simulink model "Grid_SensorLayout_SpatialAllignment_Clustering"  (R2018a)
settings: Solver=FixedStepAuto  StartTime=0.0  StopTime=SimulationTime  FixedStep=SamplingTime  RelTol=1e-3
values from neighbouring files (symbols this model uses):
  ValidateGRID = true    [SensorFusion_Script0_main.m]
  ValidateLAYOUT = true    [SensorFusion_Script0_main.m]
  VisualizeCLUSTERING = true    [SensorFusion_Script0_main.m]
undefined symbols (not defined in the file or in its folder): ACTIVATE_CAM, ACTIVATE_RAD, CAM1_detTimeStamp, CAM1_MeasNoise, CAM1_objClassID, CAM1_PX, CAM1_PY, CAM1_VX, CAM1_VY, CAM2_detTimeStamp, CAM2_MeasNoise, CAM2_objClassID, CAM2_PX, CAM2_PY, CAM2_VX, CAM2_VY, CAM3_detTimeStamp, CAM3_MeasNoise, CAM3_objClassID, CAM3_PX, CAM3_PY, CAM3_VX, CAM3_VY, CAM4_detTimeStamp, CAM4_MeasNoise, CAM4_objClassID, CAM4_PX, CAM4_PY, CAM4_VX, CAM4_VY, CAM5_detTimeStamp, CAM5_MeasNoise, CAM5_objClassID, CAM5_PX, CAM5_PY, CAM5_VX, CAM5_VY, CAM6_detTimeStamp, CAM6_MeasNoise, CAM6_objClassID, CAM6_PX, CAM6_PY, CAM6_VX, CAM6_VY, CAM7_detTimeStamp, CAM7_MeasNoise, CAM7_objClassID, CAM7_PX, CAM7_PY, CAM7_VX, CAM7_VY, CAM8_detTimeStamp, CAM8_MeasNoise, CAM8_objClassID, CAM8_PX, CAM8_PY, CAM8_VX, CAM8_VY, CAM_nMeas, CAM_TYPE ... (+171)
libraries: simulink_extras x4
(part 5 of 10)

== system Grid_SensorLayout_SpatialAllignment_Clustering/SENSOR_MEASUREMENTS/RADAR_CAMERA_EGO_SENSOR_INTERFACE/CameraSensors/Camera5/ExtractMeasParam1 ==
  idx : Inport
  time : Inport  Port=2
  Constant : Constant  Value=CAM5_PX
  Constant1 : Constant  Value=CAM5_PY
  Constant2 : Constant  Value=CAM5_VX
  Constant3 : Constant  Value=CAM5_VY
  Constant4 : Constant  Value=CAM5_objClassID
  Constant5 : Constant  Value=CAM5_MeasNoise
  Constant6 : Constant  Value=CAM5_detTimeStamp
  Data Type Conversion : DataTypeConversion  OutDataTypeStr=int16
  MeasNoise : Selector  NumberOfDimensions=4  InputPortWidth=3  IndexOptions=Index vector (port),Select all,Select all,Index vector (port)  Indices=[1 3],1,1,1  OutputSizes=1,1,1,1
  PosX : Selector  NumberOfDimensions=2  InputPortWidth=3  IndexOptions=Index vector (port),Index vector (port)  Indices=[1 3],1  OutputSizes=1,1
  PosY : Selector  NumberOfDimensions=2  InputPortWidth=3  IndexOptions=Index vector (port),Index vector (port)  Indices=[1 3],1  OutputSizes=1,1
  Reshape : Reshape  OutputDimensionality=Customize  OutputDimensions=[4,4]
  VelX : Selector  NumberOfDimensions=2  InputPortWidth=3  IndexOptions=Index vector (port),Index vector (port)  Indices=[1 3],1  OutputSizes=1,1
  VelY : Selector  NumberOfDimensions=2  InputPortWidth=3  IndexOptions=Index vector (port),Index vector (port)  Indices=[1 3],1  OutputSizes=1,1
  snr : Selector  NumberOfDimensions=2  InputPortWidth=3  IndexOptions=Index vector (port),Index vector (port)  Indices=[1 3],1  OutputSizes=1,1
  timeStamp : Selector  NumberOfDimensions=2  InputPortWidth=3  IndexOptions=Select all,Index vector (port)  Indices=[1 3],1  OutputSizes=1,1
  PX : Outport
  PY : Outport  Port=2
  VX : Outport  Port=3
  VY : Outport  Port=4
  OBJ_TYPE : Outport  Port=5
  NOISE_COV : Outport  Port=6
  measCaptureTime : Outport  Port=7
  wires:
  Constant3/1 -> VelY/1
  Constant2/1 -> VelX/1
  VelY/1 -> VY/1
  Constant/1 -> PosX/1
  idx/1 -> MeasNoise/3, snr/3, VelY/3, VelX/3, PosY/3, PosX/3
  Constant1/1 -> PosY/1
  VelX/1 -> VX/1
  PosX/1 -> PX/1
  PosY/1 -> PY/1
  time/1 -> timeStamp/2, MeasNoise/2, snr/2, VelY/2, VelX/2, PosY/2, PosX/2
  Constant4/1 -> snr/1
  snr/1 -> Data Type Conversion/1
  Constant5/1 -> MeasNoise/1
  Constant6/1 -> timeStamp/1
  MeasNoise/1 -> Reshape/1
  timeStamp/1 -> measCaptureTime/1
  Reshape/1 -> NOISE_COV/1
  Data Type Conversion/1 -> OBJ_TYPE/1

== system Grid_SensorLayout_SpatialAllignment_Clustering/SENSOR_MEASUREMENTS/RADAR_CAMERA_EGO_SENSOR_INTERFACE/CameraSensors/Camera5/IsValid2 ==
  idx : Inport
  px : Inport  Port=2
  py : Inport  Port=3
  vx : Inport  Port=4
  vy : Inport  Port=5
  Abs{,1..3} (4 alike) : Abs
  Add : Sum  Inputs=++++
  Constant : Constant  Value=uint16(0)
  Data Type Conversion : DataTypeConversion  OutDataTypeStr=uint16
  Switch : Switch  Threshold=0.0001
  ID : Outport
  wires:
  Add/1 -> Switch/2
  Abs2/1 -> Add/3
  Constant/1 -> Switch/3
  Abs/1 -> Add/1
  px/1 -> Abs/1
  Abs3/1 -> Add/4
  Abs1/1 -> Add/2
  vy/1 -> Abs3/1
  py/1 -> Abs1/1
  vx/1 -> Abs2/1
  idx/1 -> Data Type Conversion/1
  Switch/1 -> ID/1
  Data Type Conversion/1 -> Switch/1

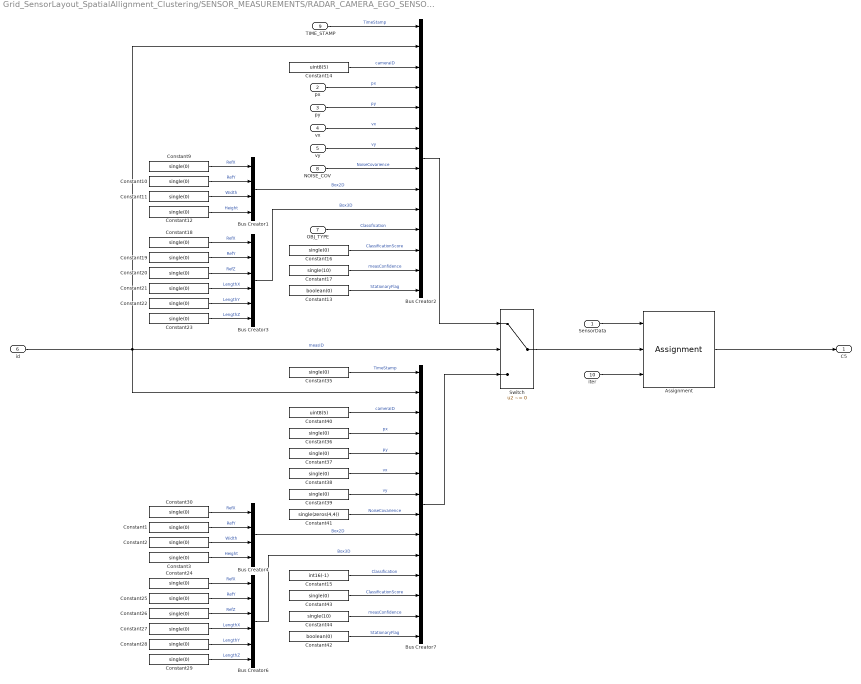
== system Grid_SensorLayout_SpatialAllignment_Clustering/SENSOR_MEASUREMENTS/RADAR_CAMERA_EGO_SENSOR_INTERFACE/CameraSensors/Camera5/Subsystem1 ==
  SensorData : Inport
  px : Inport  Port=2
  py : Inport  Port=3
  vx : Inport  Port=4
  vy : Inport  Port=5
  id : Inport  Port=6
  OBJ_TYPE : Inport  Port=7
  NOISE_COV : Inport  Port=8
  TIME_STAMP : Inport  Port=9
  iter : Inport  Port=10
  Assignment : Assignment  DiagnosticForDimensions=Warning  IndexOptions=Index vector (port)  Indices=1  OutputSizes=1
  Bus Creator1 : BusCreator  Inputs=4  OutDataTypeStr=Bus: BoxParam2D  NonVirtualBus=on
  Bus Creator2 : BusCreator  Inputs=14  OutDataTypeStr=Bus: CameraMeasParam  NonVirtualBus=on
  Bus Creator3 : BusCreator  Inputs=6  OutDataTypeStr=Bus: BoxParam3D  NonVirtualBus=on
  Bus Creator4 : BusCreator  Inputs=4  OutDataTypeStr=Bus: BoxParam2D  NonVirtualBus=on
  Bus Creator6 : BusCreator  Inputs=6  OutDataTypeStr=Bus: BoxParam3D  NonVirtualBus=on
  Bus Creator7 : BusCreator  Inputs=14  OutDataTypeStr=Bus: CameraMeasParam  NonVirtualBus=on
  Constant{1..3,9..12,16,18..30,35..39,43} (27 alike) : Constant  Value=single(0)
  Constant13 : Constant  Value=boolean(0)
  Constant14 : Constant  Value=uint8(5)
  Constant15 : Constant  Value=int16(-1)
  Constant17 : Constant  Value=single(10)
  Constant40 : Constant  Value=uint8(5)
  Constant41 : Constant  Value=single(zeros(4,4))
  Constant42 : Constant  Value=boolean(0)
  Constant44 : Constant  Value=single(10)
  Switch : Switch  Criteria=u2 ~= 0
  C5 : Outport
  wires:
  Bus Creator4/1 -> Bus Creator7/9  "Box2D"
  Bus Creator1/1 -> Bus Creator2/9  "Box2D"
  Bus Creator7/1 -> Switch/3
  Constant3/1 -> Bus Creator4/4  "Height"
  Constant44/1 -> Bus Creator7/13  "measConfidence"
  Constant19/1 -> Bus Creator3/2  "RefY"
  id/1 -> Bus Creator7/2, Bus Creator2/2, Switch/2  "measID"
  Bus Creator2/1 -> Switch/1
  Constant2/1 -> Bus Creator4/3  "Width"
  Constant12/1 -> Bus Creator1/4  "Height"
  Constant43/1 -> Bus Creator7/12  "ClassificationScore"
  Constant41/1 -> Bus Creator7/8  "NoiseCovarience"
  Constant20/1 -> Bus Creator3/3  "RefZ"
  Constant37/1 -> Bus Creator7/5  "py"
  Constant23/1 -> Bus Creator3/6  "LengthZ"
  Constant11/1 -> Bus Creator1/3  "Width"
  Constant18/1 -> Bus Creator3/1  "RefX"
  Constant9/1 -> Bus Creator1/1  "RefX"
  Constant27/1 -> Bus Creator6/4  "LengthX"
  Bus Creator3/1 -> Bus Creator2/10  "Box3D"
  Constant17/1 -> Bus Creator2/13  "measConfidence"
  py/1 -> Bus Creator2/5  "py"
  Constant36/1 -> Bus Creator7/4  "px"
  Constant16/1 -> Bus Creator2/12  "ClassificationScore"
  Constant42/1 -> Bus Creator7/14  "StationaryFlag"
  SensorData/1 -> Assignment/1
  px/1 -> Bus Creator2/4  "px"
  Constant39/1 -> Bus Creator7/7  "vy"
  Constant35/1 -> Bus Creator7/1  "TimeStamp"
  Constant38/1 -> Bus Creator7/6  "vx"
  TIME_STAMP/1 -> Bus Creator2/1  "TimeStamp"
  Switch/1 -> Assignment/2
  iter/1 -> Assignment/3
  Bus Creator6/1 -> Bus Creator7/10  "Box3D"
  Constant10/1 -> Bus Creator1/2  "RefY"
  NOISE_COV/1 -> Bus Creator2/8  "NoiseCovarience"
  Constant21/1 -> Bus Creator3/4  "LengthX"
  Constant1/1 -> Bus Creator4/2  "RefY"
  Constant25/1 -> Bus Creator6/2  "RefY"
  Constant26/1 -> Bus Creator6/3  "RefZ"
  Constant29/1 -> Bus Creator6/6  "LengthZ"
  Constant30/1 -> Bus Creator4/1  "RefX"
  vx/1 -> Bus Creator2/6  "vx"
  Constant13/1 -> Bus Creator2/14  "StationaryFlag"
  Constant22/1 -> Bus Creator3/5  "LengthY"
  Constant24/1 -> Bus Creator6/1  "RefX"
  Constant40/1 -> Bus Creator7/3  "cameraID"
  Constant28/1 -> Bus Creator6/5  "LengthY"
  Assignment/1 -> C5/1
  Constant15/1 -> Bus Creator7/11  "Classification"
  Constant14/1 -> Bus Creator2/3  "cameraID"
  vy/1 -> Bus Creator2/7  "vy"
  OBJ_TYPE/1 -> Bus Creator2/11  "Classification"

== system Grid_SensorLayout_SpatialAllignment_Clustering/SENSOR_MEASUREMENTS/RADAR_CAMERA_EGO_SENSOR_INTERFACE/CameraSensors/Camera6/ExtractMeasParam1 ==
  idx : Inport
  time : Inport  Port=2
  Constant : Constant  Value=CAM6_PX
  Constant1 : Constant  Value=CAM6_PY
  Constant2 : Constant  Value=CAM6_VX
  Constant3 : Constant  Value=CAM6_VY
  Constant4 : Constant  Value=CAM6_objClassID
  Constant5 : Constant  Value=CAM6_MeasNoise
  Constant6 : Constant  Value=CAM6_detTimeStamp
  Data Type Conversion : DataTypeConversion  OutDataTypeStr=int16
  MeasNoise : Selector  NumberOfDimensions=4  InputPortWidth=3  IndexOptions=Index vector (port),Select all,Select all,Index vector (port)  Indices=[1 3],1,1,1  OutputSizes=1,1,1,1
  PosX : Selector  NumberOfDimensions=2  InputPortWidth=3  IndexOptions=Index vector (port),Index vector (port)  Indices=[1 3],1  OutputSizes=1,1
  PosY : Selector  NumberOfDimensions=2  InputPortWidth=3  IndexOptions=Index vector (port),Index vector (port)  Indices=[1 3],1  OutputSizes=1,1
  Reshape : Reshape  OutputDimensionality=Customize  OutputDimensions=[4,4]
  VelX : Selector  NumberOfDimensions=2  InputPortWidth=3  IndexOptions=Index vector (port),Index vector (port)  Indices=[1 3],1  OutputSizes=1,1
  VelY : Selector  NumberOfDimensions=2  InputPortWidth=3  IndexOptions=Index vector (port),Index vector (port)  Indices=[1 3],1  OutputSizes=1,1
  snr : Selector  NumberOfDimensions=2  InputPortWidth=3  IndexOptions=Index vector (port),Index vector (port)  Indices=[1 3],1  OutputSizes=1,1
  timeStamp : Selector  NumberOfDimensions=2  InputPortWidth=3  IndexOptions=Select all,Index vector (port)  Indices=[1 3],1  OutputSizes=1,1
  PX : Outport
  PY : Outport  Port=2
  VX : Outport  Port=3
  VY : Outport  Port=4
  OBJ_TYPE : Outport  Port=5
  NOISE_COV : Outport  Port=6
  measCaptureTime : Outport  Port=7
  wires:
  Constant3/1 -> VelY/1
  Constant2/1 -> VelX/1
  VelY/1 -> VY/1
  Constant/1 -> PosX/1
  idx/1 -> MeasNoise/3, snr/3, VelY/3, VelX/3, PosY/3, PosX/3
  Constant1/1 -> PosY/1
  VelX/1 -> VX/1
  PosX/1 -> PX/1
  PosY/1 -> PY/1
  time/1 -> timeStamp/2, MeasNoise/2, snr/2, VelY/2, VelX/2, PosY/2, PosX/2
  Constant4/1 -> snr/1
  snr/1 -> Data Type Conversion/1
  Constant5/1 -> MeasNoise/1
  Constant6/1 -> timeStamp/1
  MeasNoise/1 -> Reshape/1
  timeStamp/1 -> measCaptureTime/1
  Reshape/1 -> NOISE_COV/1
  Data Type Conversion/1 -> OBJ_TYPE/1

== system Grid_SensorLayout_SpatialAllignment_Clustering/SENSOR_MEASUREMENTS/RADAR_CAMERA_EGO_SENSOR_INTERFACE/CameraSensors/Camera6/IsValid2 ==
  idx : Inport
  px : Inport  Port=2
  py : Inport  Port=3
  vx : Inport  Port=4
  vy : Inport  Port=5
  Abs{,1..3} (4 alike) : Abs
  Add : Sum  Inputs=++++
  Constant : Constant  Value=uint16(0)
  Data Type Conversion : DataTypeConversion  OutDataTypeStr=uint16
  Switch : Switch  Threshold=0.0001
  ID : Outport
  wires:
  Add/1 -> Switch/2
  Abs2/1 -> Add/3
  Constant/1 -> Switch/3
  Abs/1 -> Add/1
  px/1 -> Abs/1
  Abs3/1 -> Add/4
  Abs1/1 -> Add/2
  vy/1 -> Abs3/1
  py/1 -> Abs1/1
  vx/1 -> Abs2/1
  idx/1 -> Data Type Conversion/1
  Switch/1 -> ID/1
  Data Type Conversion/1 -> Switch/1

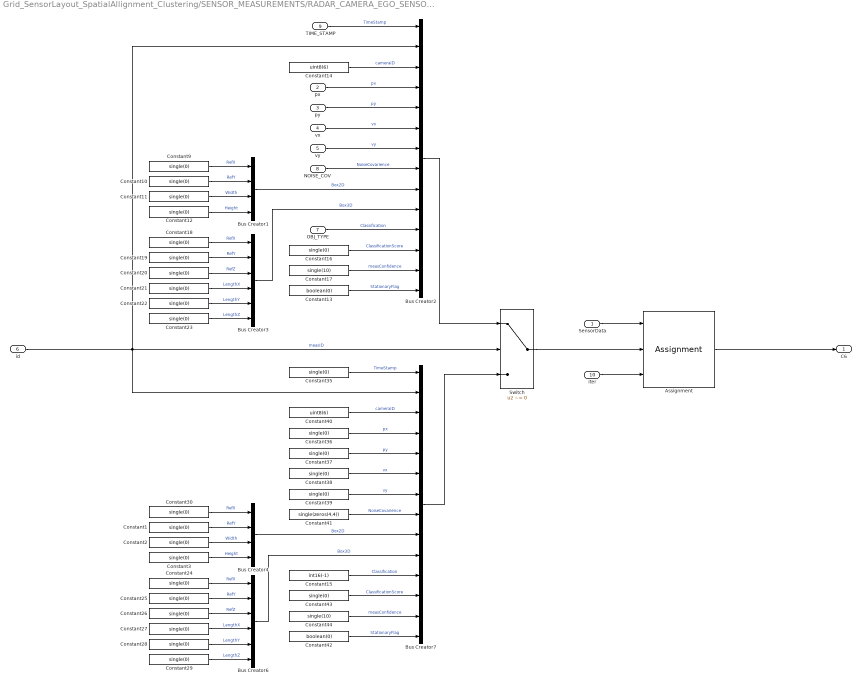
== system Grid_SensorLayout_SpatialAllignment_Clustering/SENSOR_MEASUREMENTS/RADAR_CAMERA_EGO_SENSOR_INTERFACE/CameraSensors/Camera6/Subsystem1 ==
  SensorData : Inport
  px : Inport  Port=2
  py : Inport  Port=3
  vx : Inport  Port=4
  vy : Inport  Port=5
  id : Inport  Port=6
  OBJ_TYPE : Inport  Port=7
  NOISE_COV : Inport  Port=8
  TIME_STAMP : Inport  Port=9
  iter : Inport  Port=10
  Assignment : Assignment  DiagnosticForDimensions=Warning  IndexOptions=Index vector (port)  Indices=1  OutputSizes=1
  Bus Creator1 : BusCreator  Inputs=4  OutDataTypeStr=Bus: BoxParam2D  NonVirtualBus=on
  Bus Creator2 : BusCreator  Inputs=14  OutDataTypeStr=Bus: CameraMeasParam  NonVirtualBus=on
  Bus Creator3 : BusCreator  Inputs=6  OutDataTypeStr=Bus: BoxParam3D  NonVirtualBus=on
  Bus Creator4 : BusCreator  Inputs=4  OutDataTypeStr=Bus: BoxParam2D  NonVirtualBus=on
  Bus Creator6 : BusCreator  Inputs=6  OutDataTypeStr=Bus: BoxParam3D  NonVirtualBus=on
  Bus Creator7 : BusCreator  Inputs=14  OutDataTypeStr=Bus: CameraMeasParam  NonVirtualBus=on
  Constant{1..3,9..12,16,18..30,35..39,43} (27 alike) : Constant  Value=single(0)
  Constant13 : Constant  Value=boolean(0)
  Constant14 : Constant  Value=uint8(6)
  Constant15 : Constant  Value=int16(-1)
  Constant17 : Constant  Value=single(10)
  Constant40 : Constant  Value=uint8(6)
  Constant41 : Constant  Value=single(zeros(4,4))
  Constant42 : Constant  Value=boolean(0)
  Constant44 : Constant  Value=single(10)
  Switch : Switch  Criteria=u2 ~= 0
  C6 : Outport
  wires:
  Bus Creator4/1 -> Bus Creator7/9  "Box2D"
  Bus Creator1/1 -> Bus Creator2/9  "Box2D"
  Bus Creator7/1 -> Switch/3
  Constant3/1 -> Bus Creator4/4  "Height"
  Constant44/1 -> Bus Creator7/13  "measConfidence"
  Constant19/1 -> Bus Creator3/2  "RefY"
  id/1 -> Bus Creator7/2, Bus Creator2/2, Switch/2  "measID"
  Bus Creator2/1 -> Switch/1
  Constant2/1 -> Bus Creator4/3  "Width"
  Constant12/1 -> Bus Creator1/4  "Height"
  Constant43/1 -> Bus Creator7/12  "ClassificationScore"
  Constant41/1 -> Bus Creator7/8  "NoiseCovarience"
  Constant20/1 -> Bus Creator3/3  "RefZ"
  Constant37/1 -> Bus Creator7/5  "py"
  Constant23/1 -> Bus Creator3/6  "LengthZ"
  Constant11/1 -> Bus Creator1/3  "Width"
  Constant18/1 -> Bus Creator3/1  "RefX"
  Constant9/1 -> Bus Creator1/1  "RefX"
  Constant27/1 -> Bus Creator6/4  "LengthX"
  Bus Creator3/1 -> Bus Creator2/10  "Box3D"
  Constant17/1 -> Bus Creator2/13  "measConfidence"
  py/1 -> Bus Creator2/5  "py"
  Constant36/1 -> Bus Creator7/4  "px"
  Constant16/1 -> Bus Creator2/12  "ClassificationScore"
  Constant42/1 -> Bus Creator7/14  "StationaryFlag"
  SensorData/1 -> Assignment/1
  px/1 -> Bus Creator2/4  "px"
  Constant39/1 -> Bus Creator7/7  "vy"
  Constant35/1 -> Bus Creator7/1  "TimeStamp"
  Constant38/1 -> Bus Creator7/6  "vx"
  TIME_STAMP/1 -> Bus Creator2/1  "TimeStamp"
  Switch/1 -> Assignment/2
  iter/1 -> Assignment/3
  Bus Creator6/1 -> Bus Creator7/10  "Box3D"
  Constant10/1 -> Bus Creator1/2  "RefY"
  NOISE_COV/1 -> Bus Creator2/8  "NoiseCovarience"
  Constant21/1 -> Bus Creator3/4  "LengthX"
  Constant1/1 -> Bus Creator4/2  "RefY"
  Constant25/1 -> Bus Creator6/2  "RefY"
  Constant26/1 -> Bus Creator6/3  "RefZ"
  Constant29/1 -> Bus Creator6/6  "LengthZ"
  Constant30/1 -> Bus Creator4/1  "RefX"
  vx/1 -> Bus Creator2/6  "vx"
  Constant13/1 -> Bus Creator2/14  "StationaryFlag"
  Constant22/1 -> Bus Creator3/5  "LengthY"
  Constant24/1 -> Bus Creator6/1  "RefX"
  Constant40/1 -> Bus Creator7/3  "cameraID"
  Constant28/1 -> Bus Creator6/5  "LengthY"
  Assignment/1 -> C6/1
  Constant15/1 -> Bus Creator7/11  "Classification"
  Constant14/1 -> Bus Creator2/3  "cameraID"
  vy/1 -> Bus Creator2/7  "vy"
  OBJ_TYPE/1 -> Bus Creator2/11  "Classification"

== system Grid_SensorLayout_SpatialAllignment_Clustering/SENSOR_MEASUREMENTS/RADAR_CAMERA_EGO_SENSOR_INTERFACE/CameraSensors/Camera7/ExtractMeasParam1 ==
  idx : Inport
  time : Inport  Port=2
  Constant : Constant  Value=CAM7_PX
  Constant1 : Constant  Value=CAM7_PY
  Constant2 : Constant  Value=CAM7_VX
  Constant3 : Constant  Value=CAM7_VY
  Constant4 : Constant  Value=CAM7_objClassID
  Constant5 : Constant  Value=CAM7_MeasNoise
  Constant6 : Constant  Value=CAM7_detTimeStamp
  Data Type Conversion : DataTypeConversion  OutDataTypeStr=int16
  MeasNoise : Selector  NumberOfDimensions=4  InputPortWidth=3  IndexOptions=Index vector (port),Select all,Select all,Index vector (port)  Indices=[1 3],1,1,1  OutputSizes=1,1,1,1
  PosX : Selector  NumberOfDimensions=2  InputPortWidth=3  IndexOptions=Index vector (port),Index vector (port)  Indices=[1 3],1  OutputSizes=1,1
  PosY : Selector  NumberOfDimensions=2  InputPortWidth=3  IndexOptions=Index vector (port),Index vector (port)  Indices=[1 3],1  OutputSizes=1,1
  Reshape : Reshape  OutputDimensionality=Customize  OutputDimensions=[4,4]
  VelX : Selector  NumberOfDimensions=2  InputPortWidth=3  IndexOptions=Index vector (port),Index vector (port)  Indices=[1 3],1  OutputSizes=1,1
  VelY : Selector  NumberOfDimensions=2  InputPortWidth=3  IndexOptions=Index vector (port),Index vector (port)  Indices=[1 3],1  OutputSizes=1,1
  snr : Selector  NumberOfDimensions=2  InputPortWidth=3  IndexOptions=Index vector (port),Index vector (port)  Indices=[1 3],1  OutputSizes=1,1
  timeStamp : Selector  NumberOfDimensions=2  InputPortWidth=3  IndexOptions=Select all,Index vector (port)  Indices=[1 3],1  OutputSizes=1,1
  PX : Outport
  PY : Outport  Port=2
  VX : Outport  Port=3
  VY : Outport  Port=4
  OBJ_TYPE : Outport  Port=5
  NOISE_COV : Outport  Port=6
  measCaptureTime : Outport  Port=7
  wires:
  Constant3/1 -> VelY/1
  Constant2/1 -> VelX/1
  VelY/1 -> VY/1
  Constant/1 -> PosX/1
  idx/1 -> MeasNoise/3, snr/3, VelY/3, VelX/3, PosY/3, PosX/3
  Constant1/1 -> PosY/1
  VelX/1 -> VX/1
  PosX/1 -> PX/1
  PosY/1 -> PY/1
  time/1 -> timeStamp/2, MeasNoise/2, snr/2, VelY/2, VelX/2, PosY/2, PosX/2
  Constant4/1 -> snr/1
  snr/1 -> Data Type Conversion/1
  Constant5/1 -> MeasNoise/1
  Constant6/1 -> timeStamp/1
  MeasNoise/1 -> Reshape/1
  timeStamp/1 -> measCaptureTime/1
  Reshape/1 -> NOISE_COV/1
  Data Type Conversion/1 -> OBJ_TYPE/1

== system Grid_SensorLayout_SpatialAllignment_Clustering/SENSOR_MEASUREMENTS/RADAR_CAMERA_EGO_SENSOR_INTERFACE/CameraSensors/Camera7/IsValid2 ==
  idx : Inport
  px : Inport  Port=2
  py : Inport  Port=3
  vx : Inport  Port=4
  vy : Inport  Port=5
  Abs{,1..3} (4 alike) : Abs
  Add : Sum  Inputs=++++
  Constant : Constant  Value=uint16(0)
  Data Type Conversion : DataTypeConversion  OutDataTypeStr=uint16
  Switch : Switch  Threshold=0.0001
  ID : Outport
  wires:
  Add/1 -> Switch/2
  Abs2/1 -> Add/3
  Constant/1 -> Switch/3
  Abs/1 -> Add/1
  px/1 -> Abs/1
  Abs3/1 -> Add/4
  Abs1/1 -> Add/2
  vy/1 -> Abs3/1
  py/1 -> Abs1/1
  vx/1 -> Abs2/1
  idx/1 -> Data Type Conversion/1
  Switch/1 -> ID/1
  Data Type Conversion/1 -> Switch/1

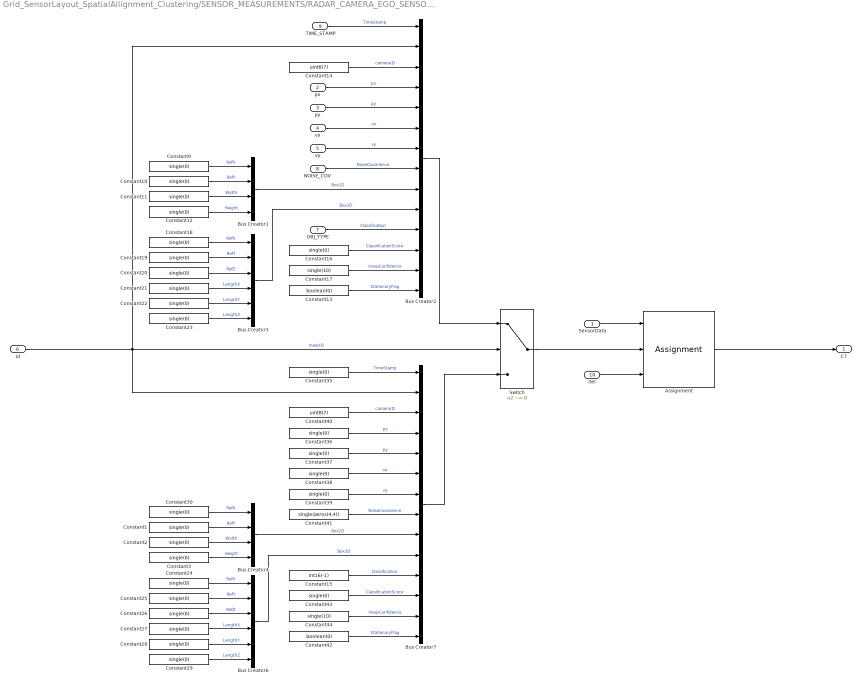
== system Grid_SensorLayout_SpatialAllignment_Clustering/SENSOR_MEASUREMENTS/RADAR_CAMERA_EGO_SENSOR_INTERFACE/CameraSensors/Camera7/Subsystem1 ==
  SensorData : Inport
  px : Inport  Port=2
  py : Inport  Port=3
  vx : Inport  Port=4
  vy : Inport  Port=5
  id : Inport  Port=6
  OBJ_TYPE : Inport  Port=7
  NOISE_COV : Inport  Port=8
  TIME_STAMP : Inport  Port=9
  iter : Inport  Port=10
  Assignment : Assignment  DiagnosticForDimensions=Warning  IndexOptions=Index vector (port)  Indices=1  OutputSizes=1
  Bus Creator1 : BusCreator  Inputs=4  OutDataTypeStr=Bus: BoxParam2D  NonVirtualBus=on
  Bus Creator2 : BusCreator  Inputs=14  OutDataTypeStr=Bus: CameraMeasParam  NonVirtualBus=on
  Bus Creator3 : BusCreator  Inputs=6  OutDataTypeStr=Bus: BoxParam3D  NonVirtualBus=on
  Bus Creator4 : BusCreator  Inputs=4  OutDataTypeStr=Bus: BoxParam2D  NonVirtualBus=on
  Bus Creator6 : BusCreator  Inputs=6  OutDataTypeStr=Bus: BoxParam3D  NonVirtualBus=on
  Bus Creator7 : BusCreator  Inputs=14  OutDataTypeStr=Bus: CameraMeasParam  NonVirtualBus=on
  Constant{1..3,9..12,16,18..30,35..39,43} (27 alike) : Constant  Value=single(0)
  Constant13 : Constant  Value=boolean(0)
  Constant14 : Constant  Value=uint8(7)
  Constant15 : Constant  Value=int16(-1)
  Constant17 : Constant  Value=single(10)
  Constant40 : Constant  Value=uint8(7)
  Constant41 : Constant  Value=single(zeros(4,4))
  Constant42 : Constant  Value=boolean(0)
  Constant44 : Constant  Value=single(10)
  Switch : Switch  Criteria=u2 ~= 0
  C7 : Outport
  wires:
  Bus Creator4/1 -> Bus Creator7/9  "Box2D"
  Bus Creator1/1 -> Bus Creator2/9  "Box2D"
  Bus Creator7/1 -> Switch/3
  Constant3/1 -> Bus Creator4/4  "Height"
  Constant44/1 -> Bus Creator7/13  "measConfidence"
  Constant19/1 -> Bus Creator3/2  "RefY"
  id/1 -> Bus Creator7/2, Bus Creator2/2, Switch/2  "measID"
  Bus Creator2/1 -> Switch/1
  Constant2/1 -> Bus Creator4/3  "Width"
  Constant12/1 -> Bus Creator1/4  "Height"
  Constant43/1 -> Bus Creator7/12  "ClassificationScore"
  Constant41/1 -> Bus Creator7/8  "NoiseCovarience"
  Constant20/1 -> Bus Creator3/3  "RefZ"
  Constant37/1 -> Bus Creator7/5  "py"
  Constant23/1 -> Bus Creator3/6  "LengthZ"
  Constant11/1 -> Bus Creator1/3  "Width"
  Constant18/1 -> Bus Creator3/1  "RefX"
  Constant9/1 -> Bus Creator1/1  "RefX"
  Constant27/1 -> Bus Creator6/4  "LengthX"
  Bus Creator3/1 -> Bus Creator2/10  "Box3D"
  Constant17/1 -> Bus Creator2/13  "measConfidence"
  py/1 -> Bus Creator2/5  "py"
  Constant36/1 -> Bus Creator7/4  "px"
  Constant16/1 -> Bus Creator2/12  "ClassificationScore"
  Constant42/1 -> Bus Creator7/14  "StationaryFlag"
  SensorData/1 -> Assignment/1
  px/1 -> Bus Creator2/4  "px"
  Constant39/1 -> Bus Creator7/7  "vy"
  Constant35/1 -> Bus Creator7/1  "TimeStamp"
  Constant38/1 -> Bus Creator7/6  "vx"
  TIME_STAMP/1 -> Bus Creator2/1  "TimeStamp"
  Switch/1 -> Assignment/2
  iter/1 -> Assignment/3
  Bus Creator6/1 -> Bus Creator7/10  "Box3D"
  Constant10/1 -> Bus Creator1/2  "RefY"
  NOISE_COV/1 -> Bus Creator2/8  "NoiseCovarience"
  Constant21/1 -> Bus Creator3/4  "LengthX"
  Constant1/1 -> Bus Creator4/2  "RefY"
  Constant25/1 -> Bus Creator6/2  "RefY"
  Constant26/1 -> Bus Creator6/3  "RefZ"
  Constant29/1 -> Bus Creator6/6  "LengthZ"
  Constant30/1 -> Bus Creator4/1  "RefX"
  vx/1 -> Bus Creator2/6  "vx"
  Constant13/1 -> Bus Creator2/14  "StationaryFlag"
  Constant22/1 -> Bus Creator3/5  "LengthY"
  Constant24/1 -> Bus Creator6/1  "RefX"
  Constant40/1 -> Bus Creator7/3  "cameraID"
  Constant28/1 -> Bus Creator6/5  "LengthY"
  Assignment/1 -> C7/1
  Constant15/1 -> Bus Creator7/11  "Classification"
  Constant14/1 -> Bus Creator2/3  "cameraID"
  vy/1 -> Bus Creator2/7  "vy"
  OBJ_TYPE/1 -> Bus Creator2/11  "Classification"

== system Grid_SensorLayout_SpatialAllignment_Clustering/SENSOR_MEASUREMENTS/RADAR_CAMERA_EGO_SENSOR_INTERFACE/CameraSensors/Camera8/ExtractMeasParam1 ==
  idx : Inport
  time : Inport  Port=2
  Constant : Constant  Value=CAM8_PX
  Constant1 : Constant  Value=CAM8_PY
  Constant2 : Constant  Value=CAM8_VX
  Constant3 : Constant  Value=CAM8_VY
  Constant4 : Constant  Value=CAM8_objClassID
  Constant5 : Constant  Value=CAM8_MeasNoise
  Constant6 : Constant  Value=CAM8_detTimeStamp
  Data Type Conversion : DataTypeConversion  OutDataTypeStr=int16
  MeasNoise : Selector  NumberOfDimensions=4  InputPortWidth=3  IndexOptions=Index vector (port),Select all,Select all,Index vector (port)  Indices=[1 3],1,1,1  OutputSizes=1,1,1,1
  PosX : Selector  NumberOfDimensions=2  InputPortWidth=3  IndexOptions=Index vector (port),Index vector (port)  Indices=[1 3],1  OutputSizes=1,1
  PosY : Selector  NumberOfDimensions=2  InputPortWidth=3  IndexOptions=Index vector (port),Index vector (port)  Indices=[1 3],1  OutputSizes=1,1
  Reshape : Reshape  OutputDimensionality=Customize  OutputDimensions=[4,4]
  VelX : Selector  NumberOfDimensions=2  InputPortWidth=3  IndexOptions=Index vector (port),Index vector (port)  Indices=[1 3],1  OutputSizes=1,1
  VelY : Selector  NumberOfDimensions=2  InputPortWidth=3  IndexOptions=Index vector (port),Index vector (port)  Indices=[1 3],1  OutputSizes=1,1
  snr : Selector  NumberOfDimensions=2  InputPortWidth=3  IndexOptions=Index vector (port),Index vector (port)  Indices=[1 3],1  OutputSizes=1,1
  timeStamp : Selector  NumberOfDimensions=2  InputPortWidth=3  IndexOptions=Select all,Index vector (port)  Indices=[1 3],1  OutputSizes=1,1
  PX : Outport
  PY : Outport  Port=2
  VX : Outport  Port=3
  VY : Outport  Port=4
  OBJ_TYPE : Outport  Port=5
  NOISE_COV : Outport  Port=6
  measCaptureTime : Outport  Port=7
  wires:
  Constant3/1 -> VelY/1
  Constant2/1 -> VelX/1
  VelY/1 -> VY/1
  Constant/1 -> PosX/1
  idx/1 -> MeasNoise/3, snr/3, VelY/3, VelX/3, PosY/3, PosX/3
  Constant1/1 -> PosY/1
  VelX/1 -> VX/1
  PosX/1 -> PX/1
  PosY/1 -> PY/1
  time/1 -> timeStamp/2, MeasNoise/2, snr/2, VelY/2, VelX/2, PosY/2, PosX/2
  Constant4/1 -> snr/1
  snr/1 -> Data Type Conversion/1
  Constant5/1 -> MeasNoise/1
  Constant6/1 -> timeStamp/1
  MeasNoise/1 -> Reshape/1
  timeStamp/1 -> measCaptureTime/1
  Reshape/1 -> NOISE_COV/1
  Data Type Conversion/1 -> OBJ_TYPE/1

== system Grid_SensorLayout_SpatialAllignment_Clustering/SENSOR_MEASUREMENTS/RADAR_CAMERA_EGO_SENSOR_INTERFACE/CameraSensors/Camera8/IsValid2 ==
  idx : Inport
  px : Inport  Port=2
  py : Inport  Port=3
  vx : Inport  Port=4
  vy : Inport  Port=5
  Abs{,1..3} (4 alike) : Abs
  Add : Sum  Inputs=++++
  Constant : Constant  Value=uint16(0)
  Data Type Conversion : DataTypeConversion  OutDataTypeStr=uint16
  Switch : Switch  Threshold=0.0001
  ID : Outport
  wires:
  Add/1 -> Switch/2
  Abs2/1 -> Add/3
  Constant/1 -> Switch/3
  Abs/1 -> Add/1
  px/1 -> Abs/1
  Abs3/1 -> Add/4
  Abs1/1 -> Add/2
  vy/1 -> Abs3/1
  py/1 -> Abs1/1
  vx/1 -> Abs2/1
  idx/1 -> Data Type Conversion/1
  Switch/1 -> ID/1
  Data Type Conversion/1 -> Switch/1

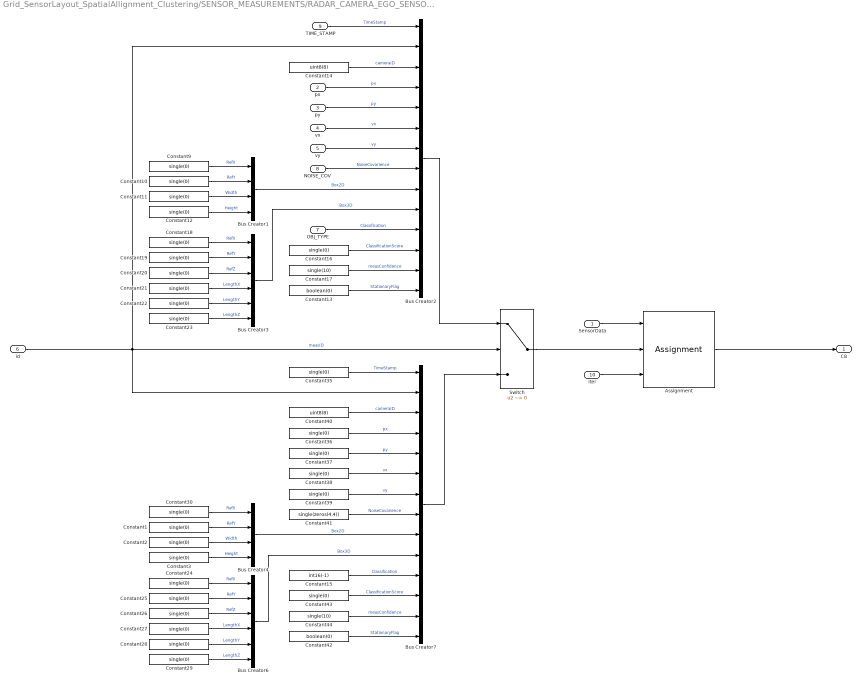
== system Grid_SensorLayout_SpatialAllignment_Clustering/SENSOR_MEASUREMENTS/RADAR_CAMERA_EGO_SENSOR_INTERFACE/CameraSensors/Camera8/Subsystem1 ==
  SensorData : Inport
  px : Inport  Port=2
  py : Inport  Port=3
  vx : Inport  Port=4
  vy : Inport  Port=5
  id : Inport  Port=6
  OBJ_TYPE : Inport  Port=7
  NOISE_COV : Inport  Port=8
  TIME_STAMP : Inport  Port=9
  iter : Inport  Port=10
  Assignment : Assignment  DiagnosticForDimensions=Warning  IndexOptions=Index vector (port)  Indices=1  OutputSizes=1
  Bus Creator1 : BusCreator  Inputs=4  OutDataTypeStr=Bus: BoxParam2D  NonVirtualBus=on
  Bus Creator2 : BusCreator  Inputs=14  OutDataTypeStr=Bus: CameraMeasParam  NonVirtualBus=on
  Bus Creator3 : BusCreator  Inputs=6  OutDataTypeStr=Bus: BoxParam3D  NonVirtualBus=on
  Bus Creator4 : BusCreator  Inputs=4  OutDataTypeStr=Bus: BoxParam2D  NonVirtualBus=on
  Bus Creator6 : BusCreator  Inputs=6  OutDataTypeStr=Bus: BoxParam3D  NonVirtualBus=on
  Bus Creator7 : BusCreator  Inputs=14  OutDataTypeStr=Bus: CameraMeasParam  NonVirtualBus=on
  Constant{1..3,9..12,16,18..30,35..39,43} (27 alike) : Constant  Value=single(0)
  Constant13 : Constant  Value=boolean(0)
  Constant14 : Constant  Value=uint8(8)
  Constant15 : Constant  Value=int16(-1)
  Constant17 : Constant  Value=single(10)
  Constant40 : Constant  Value=uint8(8)
  Constant41 : Constant  Value=single(zeros(4,4))
  Constant42 : Constant  Value=boolean(0)
  Constant44 : Constant  Value=single(10)
  Switch : Switch  Criteria=u2 ~= 0
  C8 : Outport
  wires:
  Bus Creator4/1 -> Bus Creator7/9  "Box2D"
  Bus Creator1/1 -> Bus Creator2/9  "Box2D"
  Bus Creator7/1 -> Switch/3
  Constant3/1 -> Bus Creator4/4  "Height"
  Constant44/1 -> Bus Creator7/13  "measConfidence"
  Constant19/1 -> Bus Creator3/2  "RefY"
  id/1 -> Bus Creator7/2, Bus Creator2/2, Switch/2  "measID"
  Bus Creator2/1 -> Switch/1
  Constant2/1 -> Bus Creator4/3  "Width"
  Constant12/1 -> Bus Creator1/4  "Height"
  Constant43/1 -> Bus Creator7/12  "ClassificationScore"
  Constant41/1 -> Bus Creator7/8  "NoiseCovarience"
  Constant20/1 -> Bus Creator3/3  "RefZ"
  Constant37/1 -> Bus Creator7/5  "py"
  Constant23/1 -> Bus Creator3/6  "LengthZ"
  Constant11/1 -> Bus Creator1/3  "Width"
  Constant18/1 -> Bus Creator3/1  "RefX"
  Constant9/1 -> Bus Creator1/1  "RefX"
  Constant27/1 -> Bus Creator6/4  "LengthX"
  Bus Creator3/1 -> Bus Creator2/10  "Box3D"
  Constant17/1 -> Bus Creator2/13  "measConfidence"
  py/1 -> Bus Creator2/5  "py"
  Constant36/1 -> Bus Creator7/4  "px"
  Constant16/1 -> Bus Creator2/12  "ClassificationScore"
  Constant42/1 -> Bus Creator7/14  "StationaryFlag"
  SensorData/1 -> Assignment/1
  px/1 -> Bus Creator2/4  "px"
  Constant39/1 -> Bus Creator7/7  "vy"
  Constant35/1 -> Bus Creator7/1  "TimeStamp"
  Constant38/1 -> Bus Creator7/6  "vx"
  TIME_STAMP/1 -> Bus Creator2/1  "TimeStamp"
  Switch/1 -> Assignment/2
  iter/1 -> Assignment/3
  Bus Creator6/1 -> Bus Creator7/10  "Box3D"
  Constant10/1 -> Bus Creator1/2  "RefY"
  NOISE_COV/1 -> Bus Creator2/8  "NoiseCovarience"
  Constant21/1 -> Bus Creator3/4  "LengthX"
  Constant1/1 -> Bus Creator4/2  "RefY"
  Constant25/1 -> Bus Creator6/2  "RefY"
  Constant26/1 -> Bus Creator6/3  "RefZ"
  Constant29/1 -> Bus Creator6/6  "LengthZ"
  Constant30/1 -> Bus Creator4/1  "RefX"
  vx/1 -> Bus Creator2/6  "vx"
  Constant13/1 -> Bus Creator2/14  "StationaryFlag"
  Constant22/1 -> Bus Creator3/5  "LengthY"
  Constant24/1 -> Bus Creator6/1  "RefX"
  Constant40/1 -> Bus Creator7/3  "cameraID"
  Constant28/1 -> Bus Creator6/5  "LengthY"
  Assignment/1 -> C8/1
  Constant15/1 -> Bus Creator7/11  "Classification"
  Constant14/1 -> Bus Creator2/3  "cameraID"
  vy/1 -> Bus Creator2/7  "vy"
  OBJ_TYPE/1 -> Bus Creator2/11  "Classification"

== system Grid_SensorLayout_SpatialAllignment_Clustering/SENSOR_MEASUREMENTS/RADAR_CAMERA_EGO_SENSOR_INTERFACE/RadarSensors/Radar1/CHECK_IF_DATA_VALID ==
  idx : Inport
  px : Inport  Port=2
  py : Inport  Port=3
  vx : Inport  Port=4
  vy : Inport  Port=5
  Abs{,1..3} (4 alike) : Abs
  Add : Sum  Inputs=++++
  Constant : Constant  Value=uint16(0)
  Data Type Conversion : DataTypeConversion  OutDataTypeStr=uint16
  Switch : Switch  Criteria=u2 ~= 0  Threshold=0.0001
  ID : Outport
  wires:
  Add/1 -> Switch/2
  Abs2/1 -> Add/3
  Constant/1 -> Switch/3
  Abs/1 -> Add/1
  px/1 -> Abs/1
  Abs3/1 -> Add/4
  Abs1/1 -> Add/2
  vy/1 -> Abs3/1
  py/1 -> Abs1/1
  vx/1 -> Abs2/1
  idx/1 -> Data Type Conversion/1
  Switch/1 -> ID/1
  Data Type Conversion/1 -> Switch/1

== system Grid_SensorLayout_SpatialAllignment_Clustering/SENSOR_MEASUREMENTS/RADAR_CAMERA_EGO_SENSOR_INTERFACE/RadarSensors/Radar1/GET_DATA ==
  idx : Inport
  time : Inport  Port=2
  Constant : Constant  Value=RAD1_PX
  Constant1 : Constant  Value=RAD1_PY
  Constant2 : Constant  Value=RAD1_VX
  Constant3 : Constant  Value=RAD1_VY
  Constant4 : Constant  Value=RAD1_SNR
  Constant5 : Constant  Value=RAD1_MeasNoise
  Constant6 : Constant  Value=RAD1_detTimeStamp
  MeasNoise : Selector  NumberOfDimensions=4  InputPortWidth=3  IndexOptions=Index vector (port),Select all,Select all,Index vector (port)  Indices=[1 3],1,1,1  OutputSizes=1,1,1,1
  PosX : Selector  NumberOfDimensions=2  InputPortWidth=3  IndexOptions=Index vector (port),Index vector (port)  Indices=[1 3],1  OutputSizes=1,1
  PosY : Selector  NumberOfDimensions=2  InputPortWidth=3  IndexOptions=Index vector (port),Index vector (port)  Indices=[1 3],1  OutputSizes=1,1
  Reshape : Reshape  OutputDimensionality=Customize  OutputDimensions=[4,4]
  VelX : Selector  NumberOfDimensions=2  InputPortWidth=3  IndexOptions=Index vector (port),Index vector (port)  Indices=[1 3],1  OutputSizes=1,1
  VelY : Selector  NumberOfDimensions=2  InputPortWidth=3  IndexOptions=Index vector (port),Index vector (port)  Indices=[1 3],1  OutputSizes=1,1
  snr : Selector  NumberOfDimensions=2  InputPortWidth=3  IndexOptions=Index vector (port),Index vector (port)  Indices=[1 3],1  OutputSizes=1,1
  timeStamp : Selector  NumberOfDimensions=2  InputPortWidth=3  IndexOptions=Select all,Index vector (port)  Indices=[1 3],1  OutputSizes=1,1
  PX : Outport
  PY : Outport  Port=2
  VX : Outport  Port=3
  VY : Outport  Port=4
  SNR : Outport  Port=5
  NOISE_COV : Outport  Port=6
  measCaptureTime : Outport  Port=7
  wires:
  Constant3/1 -> VelY/1
  Constant2/1 -> VelX/1
  VelY/1 -> VY/1
  Constant/1 -> PosX/1
  idx/1 -> MeasNoise/3, snr/3, VelY/3, VelX/3, PosY/3, PosX/3
  Constant1/1 -> PosY/1
  VelX/1 -> VX/1
  PosX/1 -> PX/1
  PosY/1 -> PY/1
  time/1 -> timeStamp/2, MeasNoise/2, snr/2, VelY/2, VelX/2, PosY/2, PosX/2
  Constant4/1 -> snr/1
  snr/1 -> SNR/1
  Constant5/1 -> MeasNoise/1
  Constant6/1 -> timeStamp/1
  MeasNoise/1 -> Reshape/1
  timeStamp/1 -> measCaptureTime/1
  Reshape/1 -> NOISE_COV/1

== system Grid_SensorLayout_SpatialAllignment_Clustering/SENSOR_MEASUREMENTS/RADAR_CAMERA_EGO_SENSOR_INTERFACE/RadarSensors/Radar1/SET_DATA ==
  SensorData : Inport
  px : Inport  Port=2
  py : Inport  Port=3
  vx : Inport  Port=4
  vy : Inport  Port=5
  id : Inport  Port=6
  SNR : Inport  Port=7
  NOISE_COV : Inport  Port=8
  TIME_STAMP : Inport  Port=9
  iter : Inport  Port=10
  Assignment : Assignment  DiagnosticForDimensions=Warning  IndexOptions=Index vector (port)  Indices=1  OutputSizes=1
  Bus Creator1 : BusCreator  Inputs=12  OutDataTypeStr=Bus: RadarMeasParam  NonVirtualBus=on
  Bus Creator2 : BusCreator  Inputs=12  OutDataTypeStr=Bus: RadarMeasParam  NonVirtualBus=on
  Constant{,1..5,8} (7 alike) : Constant  Value=single(0)
  Constant10 : Constant  Value=single(zeros(4,4))
  Constant13 : Constant  Value=single(10)
  Constant14 : Constant  Value=uint8(1)
  Constant16 : Constant  Value=int16(-1)
  Constant17 : Constant  Value=boolean(0)  OutDataTypeStr=boolean
  Constant6 : Constant  Value=uint8(1)
  Constant7 : Constant  Value=int16(0)
  Constant9 : Constant  Value=boolean(0)  OutDataTypeStr=boolean
  Switch : Switch  Criteria=u2 ~= 0
  R1 : Outport
  wires:
  Switch/1 -> Assignment/2
  Bus Creator2/1 -> Switch/1
  Bus Creator1/1 -> Switch/3
  Assignment/1 -> R1/1
  Constant5/1 -> Bus Creator1/9  "SNR"
  iter/1 -> Assignment/3
  id/1 -> Bus Creator1/2, Bus Creator2/2, Switch/2  "measID"
  SensorData/1 -> Assignment/1
  Constant3/1 -> Bus Creator1/7  "vy"
  Constant2/1 -> Bus Creator1/6  "vx"
  Constant1/1 -> Bus Creator1/5  "py"
  Constant/1 -> Bus Creator1/4  "px"
  Constant6/1 -> Bus Creator1/3  "radarID"
  TIME_STAMP/1 -> Bus Creator2/1  "TimeStamp"
  Constant14/1 -> Bus Creator2/3  "radarID"
  px/1 -> Bus Creator2/4  "px"
  py/1 -> Bus Creator2/5  "py"
  vx/1 -> Bus Creator2/6  "vx"
  vy/1 -> Bus Creator2/7  "vy"
  NOISE_COV/1 -> Bus Creator2/8  "NoiseCovarience"
  SNR/1 -> Bus Creator2/9  "SNR"
  Constant17/1 -> Bus Creator2/12  "StationaryFlag"
  Constant13/1 -> Bus Creator2/11  "measConfidence"
  Constant16/1 -> Bus Creator2/10  "Classification"
  Constant9/1 -> Bus Creator1/12  "StationaryFlag"
  Constant4/1 -> Bus Creator1/11  "measConfidence"
  Constant7/1 -> Bus Creator1/10  "Classification"
  Constant8/1 -> Bus Creator1/1  "TimeStamp"
  Constant10/1 -> Bus Creator1/8  "NoiseCovarience"

== system Grid_SensorLayout_SpatialAllignment_Clustering/SENSOR_MEASUREMENTS/RADAR_CAMERA_EGO_SENSOR_INTERFACE/RadarSensors/Radar2/ExtractMeasParam ==
  idx : Inport
  time : Inport  Port=2
  Constant : Constant  Value=RAD2_PX
  Constant1 : Constant  Value=RAD2_PY
  Constant2 : Constant  Value=RAD2_VX
  Constant3 : Constant  Value=RAD2_VY
  Constant4 : Constant  Value=RAD2_SNR
  Constant5 : Constant  Value=RAD2_MeasNoise
  Constant6 : Constant  Value=RAD2_detTimeStamp
  MeasNoise : Selector  NumberOfDimensions=4  InputPortWidth=3  IndexOptions=Index vector (port),Select all,Select all,Index vector (port)  Indices=[1 3],1,1,1  OutputSizes=1,1,1,1
  PosX : Selector  NumberOfDimensions=2  InputPortWidth=3  IndexOptions=Index vector (port),Index vector (port)  Indices=[1 3],1  OutputSizes=1,1
  PosY : Selector  NumberOfDimensions=2  InputPortWidth=3  IndexOptions=Index vector (port),Index vector (port)  Indices=[1 3],1  OutputSizes=1,1
  Reshape : Reshape  OutputDimensionality=Customize  OutputDimensions=[4,4]
  VelX : Selector  NumberOfDimensions=2  InputPortWidth=3  IndexOptions=Index vector (port),Index vector (port)  Indices=[1 3],1  OutputSizes=1,1
  VelY : Selector  NumberOfDimensions=2  InputPortWidth=3  IndexOptions=Index vector (port),Index vector (port)  Indices=[1 3],1  OutputSizes=1,1
  snr : Selector  NumberOfDimensions=2  InputPortWidth=3  IndexOptions=Index vector (port),Index vector (port)  Indices=[1 3],1  OutputSizes=1,1
  timeStamp : Selector  NumberOfDimensions=2  InputPortWidth=3  IndexOptions=Select all,Index vector (port)  Indices=[1 3],1  OutputSizes=1,1
  PX : Outport
  PY : Outport  Port=2
  VX : Outport  Port=3
  VY : Outport  Port=4
  SNR : Outport  Port=5
  NOISE_COV : Outport  Port=6
  measCaptureTime : Outport  Port=7
  wires:
  Constant3/1 -> VelY/1
  Constant2/1 -> VelX/1
  VelY/1 -> VY/1
  Constant/1 -> PosX/1
  idx/1 -> MeasNoise/3, snr/3, VelY/3, VelX/3, PosY/3, PosX/3
  Constant1/1 -> PosY/1
  VelX/1 -> VX/1
  PosX/1 -> PX/1
  PosY/1 -> PY/1
  time/1 -> timeStamp/2, MeasNoise/2, snr/2, VelY/2, VelX/2, PosY/2, PosX/2
  Constant4/1 -> snr/1
  snr/1 -> SNR/1
  Constant5/1 -> MeasNoise/1
  Constant6/1 -> timeStamp/1
  MeasNoise/1 -> Reshape/1
  timeStamp/1 -> measCaptureTime/1
  Reshape/1 -> NOISE_COV/1

== system Grid_SensorLayout_SpatialAllignment_Clustering/SENSOR_MEASUREMENTS/RADAR_CAMERA_EGO_SENSOR_INTERFACE/RadarSensors/Radar2/IsValid1 ==
  idx : Inport
  px : Inport  Port=2
  py : Inport  Port=3
  vx : Inport  Port=4
  vy : Inport  Port=5
  Abs{,1..3} (4 alike) : Abs
  Add : Sum  Inputs=++++
  Constant : Constant  Value=uint16(0)
  Data Type Conversion : DataTypeConversion  OutDataTypeStr=uint16
  Switch : Switch  Criteria=u2 ~= 0  Threshold=0.0001
  ID : Outport
  wires:
  Add/1 -> Switch/2
  Abs2/1 -> Add/3
  Constant/1 -> Switch/3
  Abs/1 -> Add/1
  px/1 -> Abs/1
  Abs3/1 -> Add/4
  Abs1/1 -> Add/2
  vy/1 -> Abs3/1
  py/1 -> Abs1/1
  vx/1 -> Abs2/1
  idx/1 -> Data Type Conversion/1
  Switch/1 -> ID/1
  Data Type Conversion/1 -> Switch/1

== system Grid_SensorLayout_SpatialAllignment_Clustering/SENSOR_MEASUREMENTS/RADAR_CAMERA_EGO_SENSOR_INTERFACE/RadarSensors/Radar2/Subsystem ==
  SensorData : Inport
  px : Inport  Port=2
  py : Inport  Port=3
  vx : Inport  Port=4
  vy : Inport  Port=5
  id : Inport  Port=6
  SNR : Inport  Port=7
  NOISE_COV : Inport  Port=8
  TIME_STAMP : Inport  Port=9
  iter : Inport  Port=10
  Assignment : Assignment  DiagnosticForDimensions=Warning  IndexOptions=Index vector (port)  Indices=1  OutputSizes=1
  Bus Creator1 : BusCreator  Inputs=12  OutDataTypeStr=Bus: RadarMeasParam  NonVirtualBus=on
  Bus Creator2 : BusCreator  Inputs=12  OutDataTypeStr=Bus: RadarMeasParam  NonVirtualBus=on
  Constant{,1..5,8} (7 alike) : Constant  Value=single(0)
  Constant10 : Constant  Value=single(zeros(4,4))
  Constant13 : Constant  Value=single(10)
  Constant14 : Constant  Value=uint8(2)
  Constant16 : Constant  Value=int16(-1)
  Constant17 : Constant  Value=boolean(0)  OutDataTypeStr=boolean
  Constant6 : Constant  Value=uint8(2)
  Constant7 : Constant  Value=int16(0)
  Constant9 : Constant  Value=boolean(0)  OutDataTypeStr=boolean
  Switch : Switch  Criteria=u2 ~= 0
  R2 : Outport
  wires:
  Switch/1 -> Assignment/2
  Bus Creator2/1 -> Switch/1
  Bus Creator1/1 -> Switch/3
  Assignment/1 -> R2/1
  Constant5/1 -> Bus Creator1/9  "SNR"
  iter/1 -> Assignment/3
  id/1 -> Bus Creator1/2, Bus Creator2/2, Switch/2  "measID"
  SensorData/1 -> Assignment/1
  Constant3/1 -> Bus Creator1/7  "vy"
  Constant2/1 -> Bus Creator1/6  "vx"
  Constant1/1 -> Bus Creator1/5  "py"
  Constant/1 -> Bus Creator1/4  "px"
  Constant6/1 -> Bus Creator1/3  "radarID"
  TIME_STAMP/1 -> Bus Creator2/1  "TimeStamp"
  Constant14/1 -> Bus Creator2/3  "radarID"
  px/1 -> Bus Creator2/4  "px"
  py/1 -> Bus Creator2/5  "py"
  vx/1 -> Bus Creator2/6  "vx"
  vy/1 -> Bus Creator2/7  "vy"
  NOISE_COV/1 -> Bus Creator2/8  "NoiseCovarience"
  SNR/1 -> Bus Creator2/9  "SNR"
  Constant17/1 -> Bus Creator2/12  "StationaryFlag"
  Constant13/1 -> Bus Creator2/11  "measConfidence"
  Constant16/1 -> Bus Creator2/10  "Classification"
  Constant9/1 -> Bus Creator1/12  "StationaryFlag"
  Constant4/1 -> Bus Creator1/11  "measConfidence"
  Constant7/1 -> Bus Creator1/10  "Classification"
  Constant8/1 -> Bus Creator1/1  "TimeStamp"
  Constant10/1 -> Bus Creator1/8  "NoiseCovarience"

== system Grid_SensorLayout_SpatialAllignment_Clustering/SENSOR_MEASUREMENTS/RADAR_CAMERA_EGO_SENSOR_INTERFACE/RadarSensors/Radar3/ExtractMeasParam ==
  idx : Inport
  time : Inport  Port=2
  Constant : Constant  Value=RAD3_PX
  Constant1 : Constant  Value=RAD3_PY
  Constant2 : Constant  Value=RAD3_VX
  Constant3 : Constant  Value=RAD3_VY
  Constant4 : Constant  Value=RAD3_SNR
  Constant5 : Constant  Value=RAD3_MeasNoise
  Constant6 : Constant  Value=RAD3_detTimeStamp
  MeasNoise : Selector  NumberOfDimensions=4  InputPortWidth=3  IndexOptions=Index vector (port),Select all,Select all,Index vector (port)  Indices=[1 3],1,1,1  OutputSizes=1,1,1,1
  PosX : Selector  NumberOfDimensions=2  InputPortWidth=3  IndexOptions=Index vector (port),Index vector (port)  Indices=[1 3],1  OutputSizes=1,1
  PosY : Selector  NumberOfDimensions=2  InputPortWidth=3  IndexOptions=Index vector (port),Index vector (port)  Indices=[1 3],1  OutputSizes=1,1
  Reshape : Reshape  OutputDimensionality=Customize  OutputDimensions=[4,4]
  VelX : Selector  NumberOfDimensions=2  InputPortWidth=3  IndexOptions=Index vector (port),Index vector (port)  Indices=[1 3],1  OutputSizes=1,1
  VelY : Selector  NumberOfDimensions=2  InputPortWidth=3  IndexOptions=Index vector (port),Index vector (port)  Indices=[1 3],1  OutputSizes=1,1
  snr : Selector  NumberOfDimensions=2  InputPortWidth=3  IndexOptions=Index vector (port),Index vector (port)  Indices=[1 3],1  OutputSizes=1,1
  timeStamp : Selector  NumberOfDimensions=2  InputPortWidth=3  IndexOptions=Select all,Index vector (port)  Indices=[1 3],1  OutputSizes=1,1
  PX : Outport
  PY : Outport  Port=2
  VX : Outport  Port=3
  VY : Outport  Port=4
  SNR : Outport  Port=5
  NOISE_COV : Outport  Port=6
  measCaptureTime : Outport  Port=7
  wires:
  Constant3/1 -> VelY/1
  Constant2/1 -> VelX/1
  VelY/1 -> VY/1
  Constant/1 -> PosX/1
  idx/1 -> MeasNoise/3, snr/3, VelY/3, VelX/3, PosY/3, PosX/3
  Constant1/1 -> PosY/1
  VelX/1 -> VX/1
  PosX/1 -> PX/1
  PosY/1 -> PY/1
  time/1 -> timeStamp/2, MeasNoise/2, snr/2, VelY/2, VelX/2, PosY/2, PosX/2
  Constant4/1 -> snr/1
  snr/1 -> SNR/1
  Constant5/1 -> MeasNoise/1
  Constant6/1 -> timeStamp/1
  MeasNoise/1 -> Reshape/1
  timeStamp/1 -> measCaptureTime/1
  Reshape/1 -> NOISE_COV/1

== system Grid_SensorLayout_SpatialAllignment_Clustering/SENSOR_MEASUREMENTS/RADAR_CAMERA_EGO_SENSOR_INTERFACE/RadarSensors/Radar3/IsValid1 ==
  idx : Inport
  px : Inport  Port=2
  py : Inport  Port=3
  vx : Inport  Port=4
  vy : Inport  Port=5
  Abs{,1..3} (4 alike) : Abs
  Add : Sum  Inputs=++++
  Constant : Constant  Value=uint16(0)
  Data Type Conversion : DataTypeConversion  OutDataTypeStr=uint16
  Switch : Switch  Threshold=0.0001
  ID : Outport
  wires:
  Add/1 -> Switch/2
  Abs2/1 -> Add/3
  Constant/1 -> Switch/3
  Abs/1 -> Add/1
  px/1 -> Abs/1
  Abs3/1 -> Add/4
  Abs1/1 -> Add/2
  vy/1 -> Abs3/1
  py/1 -> Abs1/1
  vx/1 -> Abs2/1
  idx/1 -> Data Type Conversion/1
  Switch/1 -> ID/1
  Data Type Conversion/1 -> Switch/1

== system Grid_SensorLayout_SpatialAllignment_Clustering/SENSOR_MEASUREMENTS/RADAR_CAMERA_EGO_SENSOR_INTERFACE/RadarSensors/Radar3/Subsystem ==
  SensorData : Inport
  px : Inport  Port=2
  py : Inport  Port=3
  vx : Inport  Port=4
  vy : Inport  Port=5
  id : Inport  Port=6
  SNR : Inport  Port=7
  NOISE_COV : Inport  Port=8
  TIME_STAMP : Inport  Port=9
  iter : Inport  Port=10
  Assignment : Assignment  DiagnosticForDimensions=Warning  IndexOptions=Index vector (port)  Indices=1  OutputSizes=1
  Bus Creator1 : BusCreator  Inputs=12  OutDataTypeStr=Bus: RadarMeasParam  NonVirtualBus=on
  Bus Creator2 : BusCreator  Inputs=12  OutDataTypeStr=Bus: RadarMeasParam  NonVirtualBus=on
  Constant{,1..5,8} (7 alike) : Constant  Value=single(0)
  Constant10 : Constant  Value=single(zeros(4,4))
  Constant13 : Constant  Value=single(10)
  Constant14 : Constant  Value=uint8(3)
  Constant16 : Constant  Value=int16(-1)
  Constant17 : Constant  Value=boolean(0)  OutDataTypeStr=boolean
  Constant6 : Constant  Value=uint8(3)
  Constant7 : Constant  Value=int16(0)
  Constant9 : Constant  Value=boolean(0)  OutDataTypeStr=boolean
  Switch : Switch  Criteria=u2 ~= 0
  R3 : Outport
  wires:
  Switch/1 -> Assignment/2
  Bus Creator2/1 -> Switch/1
  Bus Creator1/1 -> Switch/3
  Assignment/1 -> R3/1
  Constant5/1 -> Bus Creator1/9  "SNR"
  iter/1 -> Assignment/3
  id/1 -> Bus Creator1/2, Bus Creator2/2, Switch/2  "measID"
  SensorData/1 -> Assignment/1
  Constant3/1 -> Bus Creator1/7  "vy"
  Constant2/1 -> Bus Creator1/6  "vx"
  Constant1/1 -> Bus Creator1/5  "py"
  Constant/1 -> Bus Creator1/4  "px"
  Constant6/1 -> Bus Creator1/3  "radarID"
  TIME_STAMP/1 -> Bus Creator2/1  "TimeStamp"
  Constant14/1 -> Bus Creator2/3  "radarID"
  px/1 -> Bus Creator2/4  "px"
  py/1 -> Bus Creator2/5  "py"
  vx/1 -> Bus Creator2/6  "vx"
  vy/1 -> Bus Creator2/7  "vy"
  NOISE_COV/1 -> Bus Creator2/8  "NoiseCovarience"
  SNR/1 -> Bus Creator2/9  "SNR"
  Constant17/1 -> Bus Creator2/12  "StationaryFlag"
  Constant13/1 -> Bus Creator2/11  "measConfidence"
  Constant16/1 -> Bus Creator2/10  "Classification"
  Constant9/1 -> Bus Creator1/12  "StationaryFlag"
  Constant4/1 -> Bus Creator1/11  "measConfidence"
  Constant7/1 -> Bus Creator1/10  "Classification"
  Constant8/1 -> Bus Creator1/1  "TimeStamp"
  Constant10/1 -> Bus Creator1/8  "NoiseCovarience"

== system Grid_SensorLayout_SpatialAllignment_Clustering/SENSOR_MEASUREMENTS/RADAR_CAMERA_EGO_SENSOR_INTERFACE/RadarSensors/Radar4/ExtractMeasParam ==
  idx : Inport
  time : Inport  Port=2
  Constant : Constant  Value=RAD4_PX
  Constant1 : Constant  Value=RAD4_PY
  Constant2 : Constant  Value=RAD4_VX
  Constant3 : Constant  Value=RAD4_VY
  Constant4 : Constant  Value=RAD4_SNR
  Constant5 : Constant  Value=RAD4_MeasNoise
  Constant6 : Constant  Value=RAD4_detTimeStamp
  MeasNoise : Selector  NumberOfDimensions=4  InputPortWidth=3  IndexOptions=Index vector (port),Select all,Select all,Index vector (port)  Indices=[1 3],1,1,1  OutputSizes=1,1,1,1
  PosX : Selector  NumberOfDimensions=2  InputPortWidth=3  IndexOptions=Index vector (port),Index vector (port)  Indices=[1 3],1  OutputSizes=1,1
  PosY : Selector  NumberOfDimensions=2  InputPortWidth=3  IndexOptions=Index vector (port),Index vector (port)  Indices=[1 3],1  OutputSizes=1,1
  Reshape : Reshape  OutputDimensionality=Customize  OutputDimensions=[4,4]
  VelX : Selector  NumberOfDimensions=2  InputPortWidth=3  IndexOptions=Index vector (port),Index vector (port)  Indices=[1 3],1  OutputSizes=1,1
  VelY : Selector  NumberOfDimensions=2  InputPortWidth=3  IndexOptions=Index vector (port),Index vector (port)  Indices=[1 3],1  OutputSizes=1,1
  snr : Selector  NumberOfDimensions=2  InputPortWidth=3  IndexOptions=Index vector (port),Index vector (port)  Indices=[1 3],1  OutputSizes=1,1
  timeStamp : Selector  NumberOfDimensions=2  InputPortWidth=3  IndexOptions=Select all,Index vector (port)  Indices=[1 3],1  OutputSizes=1,1
  PX : Outport
  PY : Outport  Port=2
  VX : Outport  Port=3
  VY : Outport  Port=4
  SNR : Outport  Port=5
  NOISE_COV : Outport  Port=6
  measCaptureTime : Outport  Port=7
  wires:
  Constant3/1 -> VelY/1
  Constant2/1 -> VelX/1
  VelY/1 -> VY/1
  Constant/1 -> PosX/1
  idx/1 -> MeasNoise/3, snr/3, VelY/3, VelX/3, PosY/3, PosX/3
  Constant1/1 -> PosY/1
  VelX/1 -> VX/1
  PosX/1 -> PX/1
  PosY/1 -> PY/1
  time/1 -> timeStamp/2, MeasNoise/2, snr/2, VelY/2, VelX/2, PosY/2, PosX/2
  Constant4/1 -> snr/1
  snr/1 -> SNR/1
  Constant5/1 -> MeasNoise/1
  Constant6/1 -> timeStamp/1
  MeasNoise/1 -> Reshape/1
  timeStamp/1 -> measCaptureTime/1
  Reshape/1 -> NOISE_COV/1

== system Grid_SensorLayout_SpatialAllignment_Clustering/SENSOR_MEASUREMENTS/RADAR_CAMERA_EGO_SENSOR_INTERFACE/RadarSensors/Radar4/IsValid1 ==
  idx : Inport
  px : Inport  Port=2
  py : Inport  Port=3
  vx : Inport  Port=4
  vy : Inport  Port=5
  Abs{,1..3} (4 alike) : Abs
  Add : Sum  Inputs=++++
  Constant : Constant  Value=uint16(0)
  Data Type Conversion : DataTypeConversion  OutDataTypeStr=uint16
  Switch : Switch  Threshold=0.0001
  ID : Outport
  wires:
  Add/1 -> Switch/2
  Abs2/1 -> Add/3
  Constant/1 -> Switch/3
  Abs/1 -> Add/1
  px/1 -> Abs/1
  Abs3/1 -> Add/4
  Abs1/1 -> Add/2
  vy/1 -> Abs3/1
  py/1 -> Abs1/1
  vx/1 -> Abs2/1
  idx/1 -> Data Type Conversion/1
  Switch/1 -> ID/1
  Data Type Conversion/1 -> Switch/1
